simulink library "lib_rgb"  (R2022b)
settings: Solver=VariableStepAuto  StartTime=0.0  StopTime=10.0  RelTol=1e-3
settings Model: Creator=F64236C  LastModifiedBy=F64236C

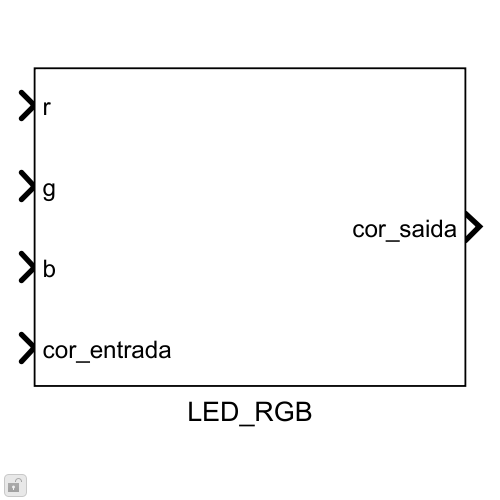
[thumbnail: Simulink's stored preview of the top-level diagram]
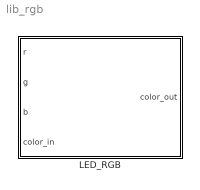
== system lib_rgb ==
  LED_RGB : Subsystem

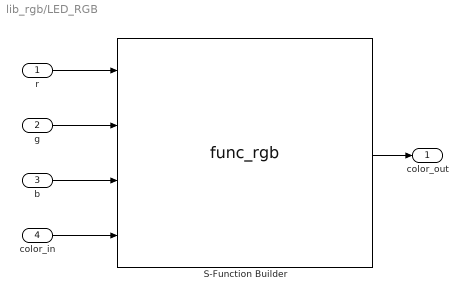
== system lib_rgb/LED_RGB ==
  r : Inport
  g : Inport  Port=2
  b : Inport  Port=3
  color_in : Inport  Port=4
  S-Function Builder : S-Function  FunctionName=func_rgb  SFunctionModules=func_rgb_wrapper.cpp  SFunctionDeploymentMode=off  EnableBusSupport=off  mask(S-Function Builder){}
      mask help: Simulink:masks:SFunctionBuilder_MD
      mask init:
      | val = [[.9  0.75 0.75 1 1 .9 .9 1]',[1 1 0.75 0.75 .9 .9 1 .9]'];try , sys = get_param(gcb,'SfunBuilderFcnName');if isempty(sys), sys = get_param(gcb,'FunctionName'); end,catch, sys = get_param(gcb,'FunctionName'); end
      settings: CopyFcn=set_param(gcbh,'LinkStatus','none')  OpenFcn=sfunctionwizard(gcbh)
      mask Display:
      | plot(val(:,1),val(:,2))
      | disp(sys)
      | port_label('input',1,'red')
      | port_label('input',2,'green')
      | port_label('input',3,'blue')
      | port_label('input',4,'color_in')
      | port_label('output',1,'color_out')
  color_out : Outport
  wires:
  color_in/1 -> S-Function Builder/4
  b/1 -> S-Function Builder/3
  r/1 -> S-Function Builder/1
  g/1 -> S-Function Builder/2
  S-Function Builder/1 -> color_out/1
